simulink model "ContactorMgmt"  (R2022b)
settings: configuration reference "BMS_Sw_CodeGenConfig" (kept outside this file)
values from neighbouring files (symbols this model uses):
  CntctWaitTime = 200    [DD_ContactorMgmt.sldd]
  PreChrgTimeOut = 1    [DD_ContactorMgmt.sldd]
  PreChrgVoltRatio = 0.95    [DD_ContactorMgmt.sldd]
undefined symbols (not defined in the file or in its folder): BMS_State_Enum, Contact
libraries: simulink x2, FaultManagement_lib x2
settings Model: DataDictionary=DD_ContactorMgmt.sldd  Creator=cpatel  LastModifiedBy=salem
settings ConfigSetRef: SourceName=BMS_Sw_CodeGenConfig

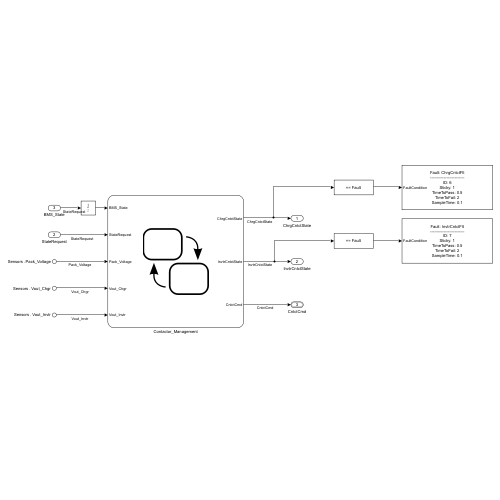
[thumbnail: Simulink's stored preview of the top-level diagram]
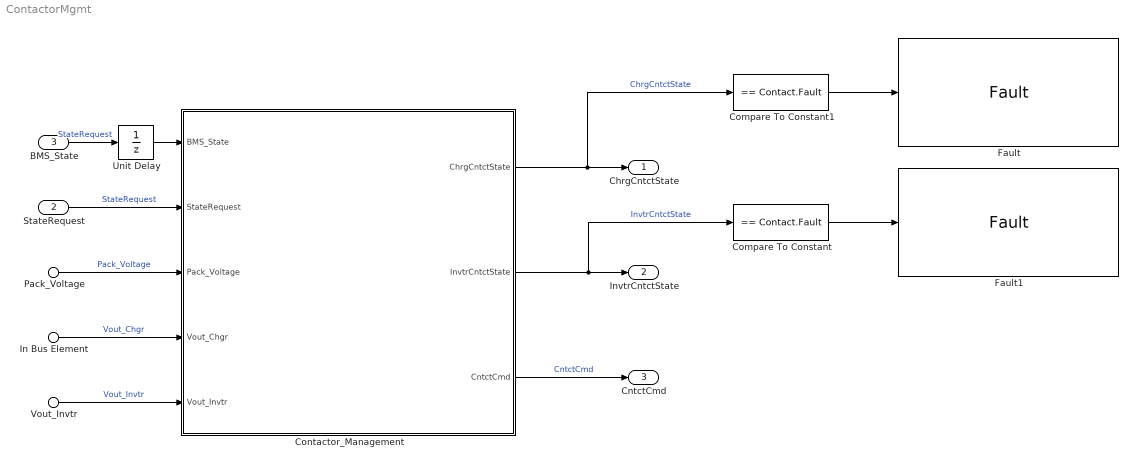
== system ContactorMgmt ==
  Pack_Voltage : Inport  PortName=Sensors  Element=Pack_Voltage
  In Bus Element : Inport  PortName=Sensors  Element=Vout_Chgr
  Vout_Invtr : Inport  PortName=Sensors  Element=Vout_Invtr
  StateRequest : Inport  Port=2  OutDataTypeStr=Enum: SRE  PortDimensions=1  SampleTime=[0.10000000000000001,0]
  BMS_State : Inport  Port=3  OutDataTypeStr=Enum: BMS_State_Enum  PortDimensions=1  SampleTime=[0.10000000000000001,0]
  Compare To Constant : simulink/Logic and Bit Operations/Compare To Constant  relop===  const=Contact.Fault  OutDataTypeStr=boolean
  Compare To Constant1 : simulink/Logic and Bit Operations/Compare To Constant  relop===  const=Contact.Fault  OutDataTypeStr=boolean
  Contactor_Management : Stateflow chart  TreatAsAtomicUnit=on  VariantControl=(default)
  Fault : FaultManagement_lib/Fault  FaultName=ChrgCntctFlt  ID=6  Enable=1  Sticky=1  TimeToFail=0.5  TimeToPass=2  SampleTime=0.1
  Fault1 : FaultManagement_lib/Fault  FaultName=InvtrCntctFlt  ID=7  Enable=1  Sticky=1  TimeToFail=0.5  TimeToPass=2  SampleTime=0.1
  Unit Delay : UnitDelay  InitialCondition=BMS_State_Enum.BMS_Standby  SampleTime=-1  HasFrameUpgradeWarning=on
  ChrgCntctState : Outport
  InvtrCntctState : Outport  Port=2
  CntctCmd : Outport  Port=3  OutDataTypeStr=Bus: CntctCmd  BusOutputAsStruct=on
  wires:
  In Bus Element/1 -> Contactor_Management/4(Vout_Chgr)  "Vout_Chgr"
  StateRequest/1 -> Contactor_Management/2(StateRequest)  "StateRequest"
  Pack_Voltage/1 -> Contactor_Management/3(Pack_Voltage)  "Pack_Voltage"
  Vout_Invtr/1 -> Contactor_Management/5(Vout_Invtr)  "Vout_Invtr"
  BMS_State/1 -> Unit Delay/1  "StateRequest"
  Contactor_Management/3(CntctCmd) -> CntctCmd/1  "CntctCmd"
  Contactor_Management/2(InvtrCntctState) -> Compare To Constant/1, InvtrCntctState/1  "InvtrCntctState"
  Contactor_Management/1(ChrgCntctState) -> Compare To Constant1/1, ChrgCntctState/1  "ChrgCntctState"
  Compare To Constant/1 -> Fault1/1
  Compare To Constant1/1 -> Fault/1
  Unit Delay/1 -> Contactor_Management/1(BMS_State)

== stateflow chart ContactorMgmt/Contactor_Management ==
  state ChrgCntctSt [parallel]
    settings: executionOrder=1
    state CloseChgrCntct
      state CloseNegCntct
        CntctCmd.NegCntctChgrCmd = true;
      state PreChrgFlt
        ChrgCntctState = Contact.Fault;
      state ClosePreChrgRly
        CntctCmd.PreChrgRelayChgrCmd = true;
      state ClosePosCntct
        CntctCmd.PosCntctChgrCmd = true;
      state OpenPreChrgRly
        CntctCmd.PreChrgRelayChgrCmd = false;
        ChrgCntctState = Contact.Close;
      (default) -> ChrgCntctSt.CloseChgrCntct.CloseNegCntct : {ChrgCntctState = Contact.Init;}
      ChrgCntctSt.CloseChgrCntct.CloseNegCntct -> ChrgCntctSt.CloseChgrCntct.ClosePreChrgRly : after(CntctWaitTime,msec)
      ChrgCntctSt.CloseChgrCntct.ClosePreChrgRly -> ChrgCntctSt.CloseChgrCntct.PreChrgFlt [order 1] : after(PreChrgTimeOut,sec)
          | % Check timeout
      ChrgCntctSt.CloseChgrCntct.ClosePreChrgRly -> ChrgCntctSt.CloseChgrCntct.ClosePosCntct [order 2] : [Vout_Chgr/Pack_Voltage >=PreChrgVoltRatio]
      ChrgCntctSt.CloseChgrCntct.ClosePosCntct -> ChrgCntctSt.CloseChgrCntct.OpenPreChrgRly : after(CntctWaitTime,msec)
    state OpenChgrCntct
      state ClosePreChrgRly
        CntctCmd.PreChrgRelayChgrCmd = true;
      state OpenPosCntct
        CntctCmd.PosCntctChgrCmd = false;
      state OpenPreChrgRly
        CntctCmd.PreChrgRelayChgrCmd = false;
      state OpenNegCntct
        CntctCmd.NegCntctChgrCmd = false;
        ChrgCntctState = Contact.Open;
      (default) -> ChrgCntctSt.OpenChgrCntct.ClosePreChrgRly : {ChrgCntctState = Contact.Init;}
      ChrgCntctSt.OpenChgrCntct.ClosePreChrgRly -> ChrgCntctSt.OpenChgrCntct.OpenPosCntct : after(CntctWaitTime,msec)
          | % Check for low current
      ChrgCntctSt.OpenChgrCntct.OpenPosCntct -> ChrgCntctSt.OpenChgrCntct.OpenPreChrgRly : after(CntctWaitTime,msec)
      ChrgCntctSt.OpenChgrCntct.OpenPreChrgRly -> ChrgCntctSt.OpenChgrCntct.OpenNegCntct : after(CntctWaitTime,msec)
    (default) -> OpenChgrCntct : {ChrgCntctState = Contact.Init;}
    CloseChgrCntct -> OpenChgrCntct : [StateRequest ~= SRE.Charging || ...
        | BMS_State == BMS_State_Enum.BMS_Fault]
    OpenChgrCntct -> CloseChgrCntct : [StateRequest == SRE.Charging && ...
        | InvtrCntctState == Contact.Open && ...
        | BMS_State ~= BMS_State_Enum.BMS_Fault]
  state InvtrCntctSt [parallel]
    settings: executionOrder=2
    state OpenInvtrCntct
      state ClosePreChrgRly
        CntctCmd.PreChrgRelayInvtrCmd = true;
      state OpenPosCntct
        CntctCmd.PosCntctInvtrCmd = false;
      state OpenPreChrgRly
        CntctCmd.PreChrgRelayInvtrCmd = false;
      state OpenNegCntct
        CntctCmd.NegCntctInvtrCmd = false;
        InvtrCntctState = Contact.Open;
      (default) -> InvtrCntctSt.OpenInvtrCntct.ClosePreChrgRly : {InvtrCntctState = Contact.Init;}
      InvtrCntctSt.OpenInvtrCntct.ClosePreChrgRly -> InvtrCntctSt.OpenInvtrCntct.OpenPosCntct : after(CntctWaitTime,msec)
          | % Check for low current
      InvtrCntctSt.OpenInvtrCntct.OpenPosCntct -> InvtrCntctSt.OpenInvtrCntct.OpenPreChrgRly : after(CntctWaitTime,msec)
      InvtrCntctSt.OpenInvtrCntct.OpenPreChrgRly -> InvtrCntctSt.OpenInvtrCntct.OpenNegCntct : after(CntctWaitTime,msec)
    state CloseInvtrCntct
      state CloseNegCntct
        CntctCmd.NegCntctInvtrCmd = true;
      state ClosePreChrgRly
        CntctCmd.PreChrgRelayInvtrCmd = true;
      state PreChrgFlt
        InvtrCntctState = Contact.Fault;
      state ClosePosCntct
        CntctCmd.PosCntctInvtrCmd = true;
      state OpenPreChrgRly
        CntctCmd.PreChrgRelayInvtrCmd = false;
        InvtrCntctState = Contact.Close;
      (default) -> InvtrCntctSt.CloseInvtrCntct.CloseNegCntct : {InvtrCntctState = Contact.Init;}
      InvtrCntctSt.CloseInvtrCntct.CloseNegCntct -> InvtrCntctSt.CloseInvtrCntct.ClosePreChrgRly : after(CntctWaitTime,msec)
      InvtrCntctSt.CloseInvtrCntct.ClosePreChrgRly -> InvtrCntctSt.CloseInvtrCntct.PreChrgFlt [order 1] : after(PreChrgTimeOut,sec)
          | % Check timeout
      InvtrCntctSt.CloseInvtrCntct.ClosePreChrgRly -> InvtrCntctSt.CloseInvtrCntct.ClosePosCntct [order 2] : [Vout_Invtr/Pack_Voltage >=PreChrgVoltRatio]
      InvtrCntctSt.CloseInvtrCntct.ClosePosCntct -> InvtrCntctSt.CloseInvtrCntct.OpenPreChrgRly : after(CntctWaitTime,msec)
    (default) -> OpenInvtrCntct : {InvtrCntctState =Contact.Init;}
    CloseInvtrCntct -> OpenInvtrCntct : [StateRequest ~= SRE.Driving || ...
        | BMS_State == BMS_State_Enum.BMS_Fault]
    OpenInvtrCntct -> CloseInvtrCntct : [StateRequest == SRE.Driving && ...
        | ChrgCntctState == Contact.Open && ...
        | BMS_State ~= BMS_State_Enum.BMS_Fault]
  data: BMS_State input; StateRequest input Enum: SRE; Pack_Voltage input single; Vout_Chgr input single; Vout_Invtr input single; CntctWaitTime parameter uint16; PreChrgTimeOut parameter uint8; PreChrgVoltRatio parameter single; ChrgCntctState output Enum: Contact; InvtrCntctState output Enum: Contact; CntctCmd output Bus: CntctCmd
